simulink model "fw_simple_mixer"  (R2024b)
settings: Solver=FixedStepAuto  StartTime=0.0  StopTime=10.0  FixedStep=0.005  RelTol=1e-3
settings Model: DataDictionary=nextpilot_datadict.sldd  Creator=CETCA  LastModifiedBy=CETCA

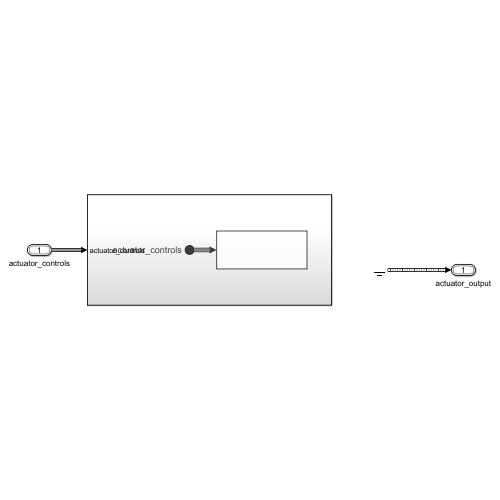
[thumbnail: Simulink's stored preview of the top-level diagram]
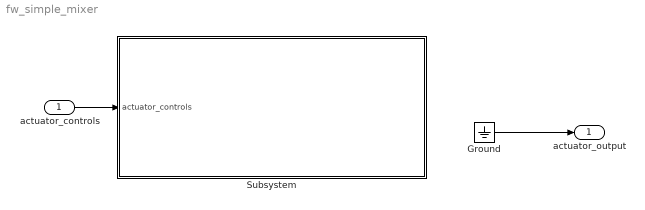
== system fw_simple_mixer ==
  actuator_controls : Inport  OutDataTypeStr=Bus: actuator_controls_s
  Ground : Ground
  Subsystem : Subsystem
  actuator_output : Outport  OutDataTypeStr=Bus: actuator_outputs_s
  wires:
  actuator_controls/1 -> Subsystem/1(actuator_controls)
  Ground/1 -> actuator_output/1

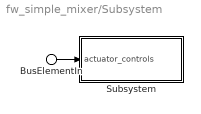
== system fw_simple_mixer/Subsystem ==
  BusElementIn : Inport  PortName=actuator_controls
  Subsystem : Subsystem
  wires:
  BusElementIn/1 -> Subsystem/1(actuator_controls)

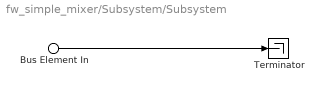
== system fw_simple_mixer/Subsystem/Subsystem ==
  Bus Element In : Inport  PortName=actuator_controls  Element=control
  Terminator : Terminator
  wires:
  Bus Element In/1 -> Terminator/1
